simulink model "rectifier_6n12pulse"  (R2014a)
settings: Solver=ode23tb  StartTime=0.0  StopTime=0.2  FixedStep=Ts  MaxStep=1e-4  RelTol=1e-4
PreLoadFcn:
  | Ts=2e-6;
InitFcn:
  | Ts=2e-6;
StartFcn:
  | tic;
StopFcn:
  | toc;
undefined symbols (not defined in the file or in its folder): C, D1, Delta
libraries: powerlib x21
settings Model: Creator=gdudgeon  LastModifiedBy=cosorio
settings DataIOCC: SignalLoggingSaveFormat=ModelDataLogs  SaveTime=off
settings OptimizationCC: ExpressionDepthLimit=2147483647  InitFltsAndDblsToZero=on
settings DebuggingCC: SaveWithParameterizedLinksMsg=none  UnderspecifiedInitializationDetection=Classic  SignalResolutionControl=TryResolveAllWithWarning  MultiTaskDSMMsg=warning  MultiTaskCondExecSysMsg=none  FcnCallInpInsideContextMsg=UseLocalSettings  StateNameClashWarn=warning
settings RTWCC: IncludeERTFirstTime=on
settings GRTTargetCC: TargetFcnLib=ansi_tfl_tmw.mat  CombineOutputUpdateFcns=off  GRTInterface=on

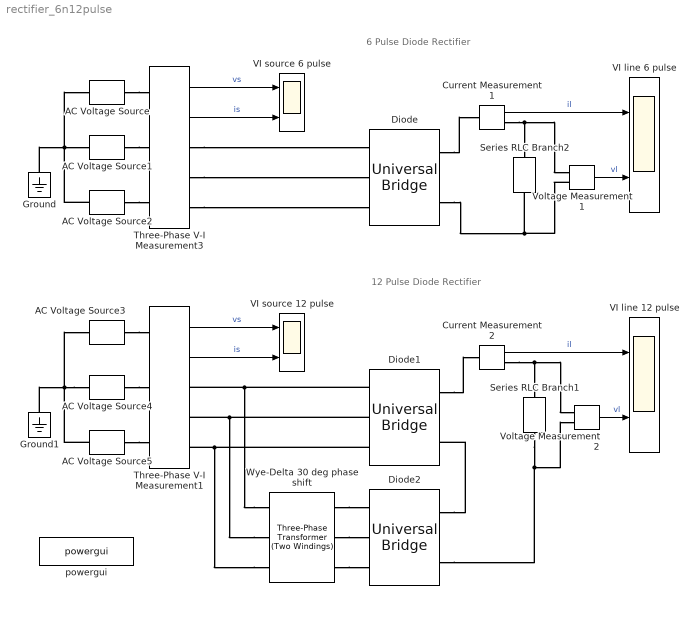
== system rectifier_6n12pulse ==
  note: 6 Pulse Diode Rectifier
  note: 12 Pulse Diode Rectifier
  AC Voltage Source : powerlib/Electrical Sources/AC Voltage Source  Amplitude=100/sqrt(3)  Phase=0  Frequency=60  SampleTime=0  Measurements=None
  AC Voltage Source1 : powerlib/Electrical Sources/AC Voltage Source  Amplitude=100/sqrt(3)  Phase=-120  Frequency=60  SampleTime=0  Measurements=None
  AC Voltage Source2 : powerlib/Electrical Sources/AC Voltage Source  Amplitude=100/sqrt(3)  Phase=120  Frequency=60  SampleTime=0  Measurements=None
  AC Voltage Source3 : powerlib/Electrical Sources/AC Voltage Source  Amplitude=100/sqrt(3)  Phase=0  Frequency=60  SampleTime=0  Measurements=None
  AC Voltage Source4 : powerlib/Electrical Sources/AC Voltage Source  Amplitude=100/sqrt(3)  Phase=-120  Frequency=60  SampleTime=0  Measurements=None
  AC Voltage Source5 : powerlib/Electrical Sources/AC Voltage Source  Amplitude=100/sqrt(3)  Phase=120  Frequency=60  SampleTime=0  Measurements=None
  Current Measurement1 : powerlib/Measurements/Current Measurement  PhasorSimulation=off  OutputType=Complex  PSBequivalent=0
  Current Measurement2 : powerlib/Measurements/Current Measurement  PhasorSimulation=off  OutputType=Complex  PSBequivalent=0
  Diode : powerlib/Power Electronics/Universal Bridge  Arms=3  SnubberResistance=1000  SnubberCapacitance=1e-6  Device=Diodes  Ron=1e-3  Lon=0  ForwardVoltages=[0 0]  ForwardVoltage=0.8  GTOparameters=[0 0]  IGBTparameters=[1e-6 2e-6]  Measurements=None  Measurements_2=None  converterType=Rectifier
  Diode1 : powerlib/Power Electronics/Universal Bridge  Arms=3  SnubberResistance=1000  SnubberCapacitance=1e-6  Device=Diodes  Ron=1e-3  Lon=0  ForwardVoltages=[0 0]  ForwardVoltage=0.8  GTOparameters=[0 0]  IGBTparameters=[1e-6 2e-6]  Measurements=None  Measurements_2=None  converterType=Rectifier
  Diode2 : powerlib/Power Electronics/Universal Bridge  Arms=3  SnubberResistance=1000  SnubberCapacitance=1e-6  Device=Diodes  Ron=1e-3  Lon=0  ForwardVoltages=[0 0]  ForwardVoltage=0.8  GTOparameters=[0 0]  IGBTparameters=[1e-6 2e-6]  Measurements=None  Measurements_2=None  converterType=Rectifier
  Ground : powerlib/Elements/Ground  LConnTagsString=a
  Ground1 : powerlib/Elements/Ground  LConnTagsString=a
  Series RLC Branch1 : powerlib/Elements/Series RLC Branch  LConnTagsString=__new0  RConnTagsString=__new0  BranchType=R  Resistance=1  Inductance=[]  SetiL0=off  InitialCurrent=0  Capacitance=C  Setx0=off  InitialVoltage=0  Measurements=None
  Series RLC Branch2 : powerlib/Elements/Series RLC Branch  LConnTagsString=__new0  RConnTagsString=__new0  BranchType=R  Resistance=1  Inductance=[]  SetiL0=off  InitialCurrent=0  Capacitance=C  Setx0=off  InitialVoltage=0  Measurements=None
  Three-Phase V-I Measurement1 : powerlib/Measurements/Three-Phase V-I Measurement  VoltageMeasurement=phase-to-phase  SetLabelV=off  LabelV=Vabc  Vpu=off  VpuLL=off  CurrentMeasurement=yes  SetLabelI=off  LabelI=Iabc  Ipu=off  Pbase=100e6  Vbase=500e3  OutputType=Complex  PhasorSimulation=off  PSBequivalent=0
  Three-Phase V-I Measurement3 : powerlib/Measurements/Three-Phase V-I Measurement  VoltageMeasurement=phase-to-phase  SetLabelV=off  LabelV=Vabc  Vpu=off  VpuLL=off  CurrentMeasurement=yes  SetLabelI=off  LabelI=Iabc  Ipu=off  Pbase=100e6  Vbase=500e3  OutputType=Complex  PhasorSimulation=off  PSBequivalent=0
  VI line 12 pulse : Scope  NumInputPorts=2
      settings: YMin=0~0  YMax=250~250  SaveName=viline12
  VI line 6 pulse : Scope  NumInputPorts=2
      settings: YMin=0~0  YMax=150~150  SaveName=viline6
  VI source 12 pulse : Scope  NumInputPorts=2
      settings: YMin=-200~-500  YMax=200~500  SaveName=visource12
  VI source 6 pulse : Scope  NumInputPorts=2
      settings: YMin=-200~-150  YMax=200~150  SaveName=visource6
  Voltage Measurement1 : powerlib/Measurements/Voltage Measurement  PhasorSimulation=off  OutputType=Complex  PSBequivalent=0
  Voltage Measurement2 : powerlib/Measurements/Voltage Measurement  PhasorSimulation=off  OutputType=Complex  PSBequivalent=0
  Wye-Delta 30 deg phase shift : powerlib/Elements/Three-Phase Transformer (Two Windings)  Winding1Connection=Y  UNITS=pu  NominalPower=[1e4 , 60 ]  Winding1=[100 , 1e-5, 1e-5]  Winding2Connection=Delta (D1)  Winding2=[ 100 , 1e-5, 1e-5]  SetSaturation=off  Rm=500  Lm=500  Saturation=[ 0,0 ; 0.0024,1.2 ; 1.0,1.52 ]  Hysteresis=off  DataFile='hysteresis'  SetInitialFlux=off  InitialFluxes=[ 0.8 , -0.8 , 0.7 ]  Measurements=None  MoreParameters=off  BreakLoop=off  DataType=off  TransfoNumber=1
  powergui : powerlib/powergui  Priority=2  SimulationMode=Continuous  SolverType=Tustin  SampleTime=Ts  frequency=60  SPID=off  DisableSnubberDevices=off  DisableRonSwitches=off  DisableVfSwitches=off  SwTol=0  Interpol=off  DisplayEquations=off  Ts=0  methode=off  frequencyindice=60  Pbase=100e6  ErrMax=1e-4  Iterations=50  UnitsV=kV  UnitsW=MW  FunctionMessages=off  echomessages=off  HookPort=off  EnableUseOfTLC=off  x0status=blocks  RestoreLinks=warning  ResistiveCurrentMeasurement=off  Frange=[0:2:500]  Ylog=off  Xlog=on  ShowGrid=off  save=off  variable=ZData  structure=visource6  ZoomFFT=off  StartTime=0.05  cycles=2  DisplayStyle=1  fundamental=60  FreqAxis=on  MaxFrequency=2000  frequencyindicesteady=1  RmsSteady=1  display=off
  wires:
  Three-Phase V-I Measurement3/1 -> VI source 6 pulse/1  "vs"
  Three-Phase V-I Measurement3/2 -> VI source 6 pulse/2  "is"
  Current Measurement1/1 -> VI line 6 pulse/1  "il"
  Three-Phase V-I Measurement1/1 -> VI source 12 pulse/1  "vs"
  Three-Phase V-I Measurement1/2 -> VI source 12 pulse/2  "is"
  Voltage Measurement2/1 -> VI line 12 pulse/2  "vl"
  Current Measurement2/1 -> VI line 12 pulse/1  "il"
  Voltage Measurement1/1 -> VI line 6 pulse/2  "vl"
  connections:
  AC Voltage Source2/LConn1 -- Ground/LConn1 -- AC Voltage Source/LConn1 -- AC Voltage Source1/LConn1
  AC Voltage Source/RConn1 -- Three-Phase V-I Measurement3/LConn1
  AC Voltage Source1/RConn1 -- Three-Phase V-I Measurement3/LConn2
  AC Voltage Source2/RConn1 -- Three-Phase V-I Measurement3/LConn3
  Three-Phase V-I Measurement3/RConn1 -- Diode/LConn1
  Three-Phase V-I Measurement3/RConn2 -- Diode/LConn2
  Three-Phase V-I Measurement3/RConn3 -- Diode/LConn3
  Current Measurement1/RConn1 -- Voltage Measurement1/LConn1 -- Series RLC Branch2/LConn1
  Diode/RConn1 -- Current Measurement1/LConn1
  Voltage Measurement1/LConn2 -- Series RLC Branch2/RConn1 -- Diode/RConn2
  AC Voltage Source4/LConn1 -- Ground1/LConn1 -- AC Voltage Source5/LConn1 -- AC Voltage Source3/LConn1
  Wye-Delta 30 deg phase shift/LConn1 -- Diode1/LConn1 -- Three-Phase V-I Measurement1/RConn1
  Wye-Delta 30 deg phase shift/LConn2 -- Diode1/LConn2 -- Three-Phase V-I Measurement1/RConn2
  Wye-Delta 30 deg phase shift/LConn3 -- Diode1/LConn3 -- Three-Phase V-I Measurement1/RConn3
  Current Measurement2/RConn1 -- Voltage Measurement2/LConn1 -- Series RLC Branch1/LConn1
  Diode2/RConn2 -- Voltage Measurement2/LConn2 -- Series RLC Branch1/RConn1
  Diode1/RConn1 -- Current Measurement2/LConn1
  AC Voltage Source4/RConn1 -- Three-Phase V-I Measurement1/LConn2
  Wye-Delta 30 deg phase shift/RConn3 -- Diode2/LConn3
  AC Voltage Source5/RConn1 -- Three-Phase V-I Measurement1/LConn3
  Diode2/RConn1 -- Diode1/RConn2
  Wye-Delta 30 deg phase shift/RConn1 -- Diode2/LConn1
  Wye-Delta 30 deg phase shift/RConn2 -- Diode2/LConn2
  AC Voltage Source3/RConn1 -- Three-Phase V-I Measurement1/LConn1
